simulink model "robocup_simu"  (R2022b)
settings: Solver=VariableStepAuto  StartTime=0.0  StopTime=10.0  RelTol=1e-3
values from neighbouring files (symbols this model uses):
  alpha_cap = 30    [Robotcup_V0.m]
  reduction_roues = 2.75    [Robotcup_V0.m]
  roues = 0.05    [Robotcup_V0.m]
  scaling = 31.42    [Robotcup_V0.m]
  Te = 0.100    (= 0.1)    [Robotcup_V0.m]
  u_max = 10    [Robotcup_V0.m]
  vcap = 3.2    [Robotcup_V0.m]
libraries: simulink x4
settings Model: Creator=arman  LastModifiedBy=arman

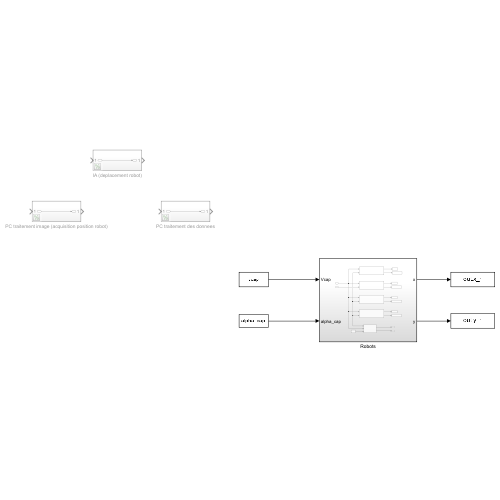
[thumbnail: Simulink's stored preview of the top-level diagram]
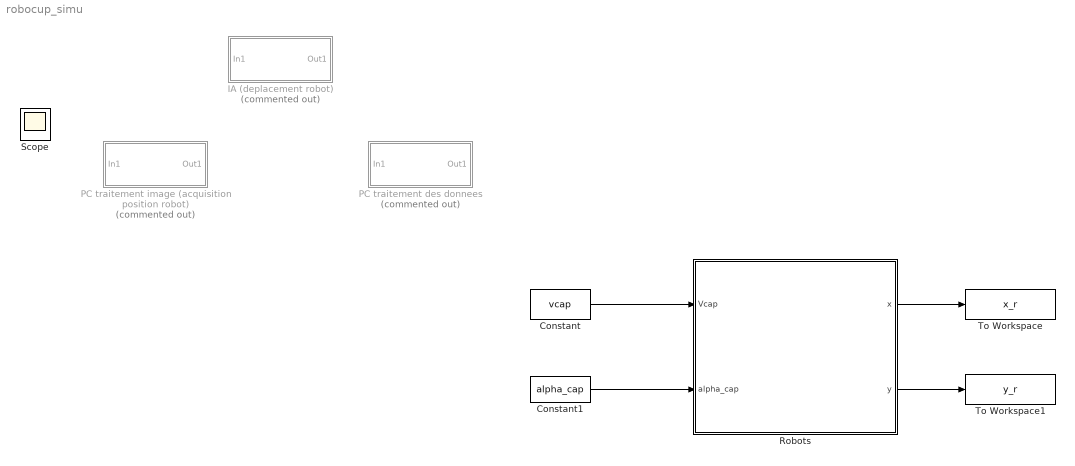
== system robocup_simu ==
  Constant : Constant  Value=vcap
  Constant1 : Constant  Value=alpha_cap
  IA (deplacement robot) : Subsystem  Commented=on
  PC traitement des donnees : Subsystem  Commented=on
  PC traitement image (acquisition position robot) : Subsystem  Commented=on
  Robots : Subsystem
  To Workspace : ToWorkspace  VariableName=x_r  SampleTime=-1
  To Workspace1 : ToWorkspace  VariableName=y_r  SaveFormat=Timeseries  SampleTime=-1
  Scope : Scope
  wires:
  Robots/1(x) -> To Workspace/1
  Robots/2(y) -> To Workspace1/1
  Constant/1 -> Robots/1(Vcap)
  Constant1/1 -> Robots/2(alpha_cap)

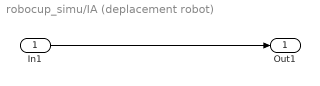
== system robocup_simu/IA (deplacement robot) ==
  In1 : Inport
  Out1 : Outport
  wires:
  In1/1 -> Out1/1

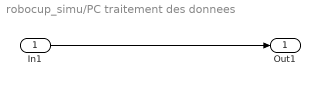
== system robocup_simu/PC traitement des donnees ==
  In1 : Inport
  Out1 : Outport
  wires:
  In1/1 -> Out1/1

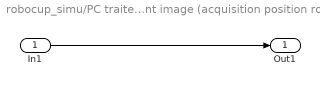
== system robocup_simu/PC traitement image (acquisition position robot) ==
  In1 : Inport
  Out1 : Outport
  wires:
  In1/1 -> Out1/1

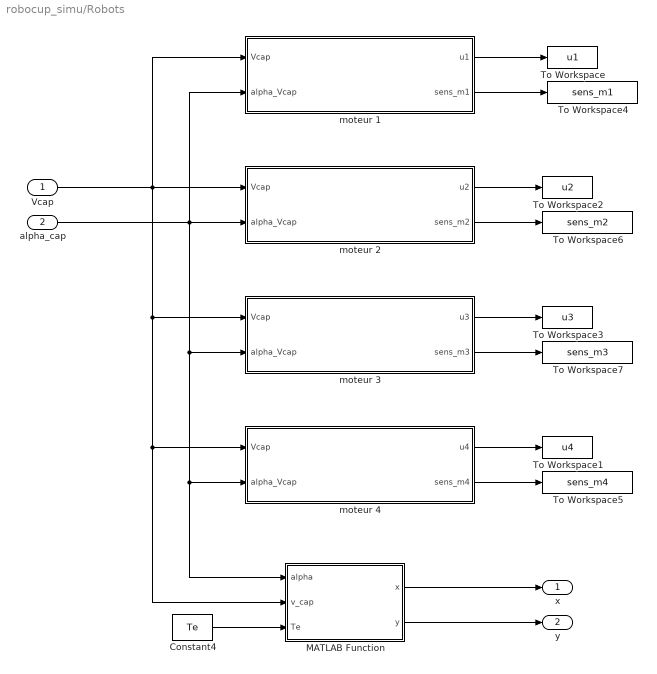
== system robocup_simu/Robots ==
  Vcap : Inport
  alpha_cap : Inport  Port=2
  Constant4 : Constant  Value=Te
  MATLAB Function : MATLAB Function  TreatAsAtomicUnit=on
  To Workspace : ToWorkspace  VariableName=u1  SaveFormat=Timeseries  SampleTime=-1
  To Workspace1 : ToWorkspace  VariableName=u4  SaveFormat=Timeseries  SampleTime=-1
  To Workspace2 : ToWorkspace  VariableName=u2  SaveFormat=Timeseries  SampleTime=-1
  To Workspace3 : ToWorkspace  VariableName=u3  SaveFormat=Timeseries  SampleTime=-1
  To Workspace4 : ToWorkspace  VariableName=sens_m1  SaveFormat=Timeseries  SampleTime=-1
  To Workspace5 : ToWorkspace  VariableName=sens_m4  SaveFormat=Timeseries  SampleTime=-1
  To Workspace6 : ToWorkspace  VariableName=sens_m2  SaveFormat=Timeseries  SampleTime=-1
  To Workspace7 : ToWorkspace  VariableName=sens_m3  SaveFormat=Timeseries  SampleTime=-1
  moteur 1 : Subsystem
  moteur 2 : Subsystem
  moteur 3 : Subsystem
  moteur 4 : Subsystem
  x : Outport
  y : Outport  Port=2
  wires:
  moteur 3/1(u3) -> To Workspace3/1
  moteur 2/1(u2) -> To Workspace2/1
  moteur 1/1(u1) -> To Workspace/1
  moteur 4/1(u4) -> To Workspace1/1
  moteur 1/2(sens_m1) -> To Workspace4/1
  moteur 3/2(sens_m3) -> To Workspace7/1
  moteur 2/2(sens_m2) -> To Workspace6/1
  moteur 4/2(sens_m4) -> To Workspace5/1
  MATLAB Function/2(y) -> y/1
  MATLAB Function/1(x) -> x/1
  Vcap/1 -> MATLAB Function/2(v_cap), moteur 4/1(Vcap), moteur 3/1(Vcap), moteur 2/1(Vcap), moteur 1/1(Vcap)
  alpha_cap/1 -> MATLAB Function/1(alpha), moteur 4/2(alpha_Vcap), moteur 3/2(alpha_Vcap), moteur 1/2(alpha_Vcap), moteur 2/2(alpha_Vcap)
  Constant4/1 -> MATLAB Function/3(Te)

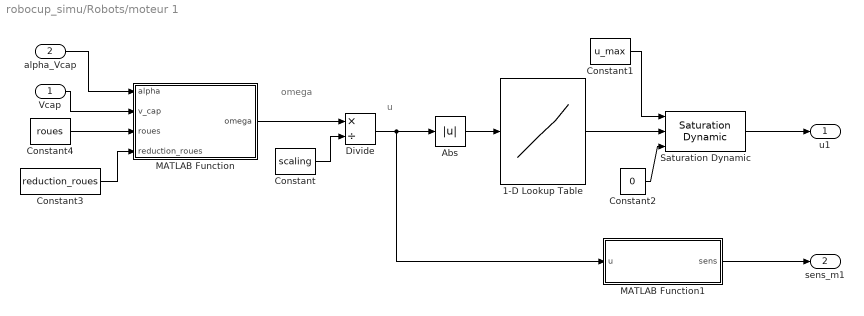
== system robocup_simu/Robots/moteur 1 ==
  note: omega
  note: u
  Vcap : Inport
  alpha_Vcap : Inport  Port=2
  1-D Lookup Table : Lookup_n-D  NumberOfTableDimensions=1  BreakpointsForDimension1=[0 0.16 0.17 0.32 0.33 1 1.5 2 3 4 10]  Table=[0 0 0.25 0.25 0.33 1 1.5 2 3 4 10]  InternalRulePriority=Speed  RndMeth=Simplest
  Abs : Abs  SaturateOnIntegerOverflow=off
  Constant : Constant  Value=scaling
  Constant1 : Constant  Value=u_max
  Constant2 : Constant  Value=0
  Constant3 : Constant  Value=reduction_roues
  Constant4 : Constant  Value=roues
  Divide : Product  Inputs=*/
  MATLAB Function : MATLAB Function  TreatAsAtomicUnit=on
  MATLAB Function1 : MATLAB Function  TreatAsAtomicUnit=on
  Saturation Dynamic : simulink/Discontinuities/Saturation Dynamic  OutMin=[]  OutMax=[]  OutDataTypeStr=Inherit: Same as second input  OutDataType=fixdt(1, 16)  OutScaling=2^-10  DoSatur=off
  u1 : Outport
  sens_m1 : Outport  Port=2
  wires:
  MATLAB Function/1(omega) -> Divide/1
  Constant/1 -> Divide/2
  Constant1/1 -> Saturation Dynamic/1
  Constant2/1 -> Saturation Dynamic/3
  Divide/1 -> MATLAB Function1/1(u), Abs/1
  Abs/1 -> 1-D Lookup Table/1
  1-D Lookup Table/1 -> Saturation Dynamic/2
  Saturation Dynamic/1 -> u1/1
  MATLAB Function1/1(sens) -> sens_m1/1
  Constant4/1 -> MATLAB Function/3(roues)
  Vcap/1 -> MATLAB Function/2(v_cap)
  Constant3/1 -> MATLAB Function/4(reduction_roues)
  alpha_Vcap/1 -> MATLAB Function/1(alpha)

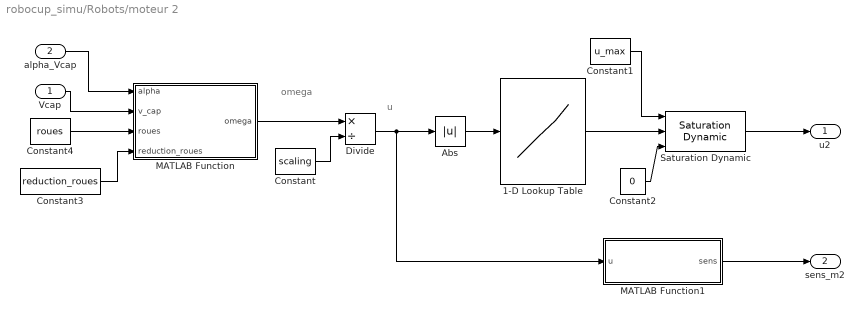
== system robocup_simu/Robots/moteur 2 ==
  note: omega
  note: u
  Vcap : Inport
  alpha_Vcap : Inport  Port=2
  1-D Lookup Table : Lookup_n-D  NumberOfTableDimensions=1  BreakpointsForDimension1=[0 0.16 0.17 0.32 0.33 1 1.5 2 3 4 10]  Table=[0 0 0.25 0.25 0.33 1 1.5 2 3 4 10]  InternalRulePriority=Speed  RndMeth=Simplest
  Abs : Abs  SaturateOnIntegerOverflow=off
  Constant : Constant  Value=scaling
  Constant1 : Constant  Value=u_max
  Constant2 : Constant  Value=0
  Constant3 : Constant  Value=reduction_roues
  Constant4 : Constant  Value=roues
  Divide : Product  Inputs=*/
  MATLAB Function : MATLAB Function  TreatAsAtomicUnit=on
  MATLAB Function1 : MATLAB Function  TreatAsAtomicUnit=on
  Saturation Dynamic : simulink/Discontinuities/Saturation Dynamic  OutMin=[]  OutMax=[]  OutDataTypeStr=Inherit: Same as second input  OutDataType=fixdt(1, 16)  OutScaling=2^-10  DoSatur=off
  u2 : Outport
  sens_m2 : Outport  Port=2
  wires:
  MATLAB Function/1(omega) -> Divide/1
  Constant/1 -> Divide/2
  Constant1/1 -> Saturation Dynamic/1
  Constant2/1 -> Saturation Dynamic/3
  Divide/1 -> MATLAB Function1/1(u), Abs/1
  Abs/1 -> 1-D Lookup Table/1
  1-D Lookup Table/1 -> Saturation Dynamic/2
  Saturation Dynamic/1 -> u2/1
  MATLAB Function1/1(sens) -> sens_m2/1
  Constant4/1 -> MATLAB Function/3(roues)
  Vcap/1 -> MATLAB Function/2(v_cap)
  Constant3/1 -> MATLAB Function/4(reduction_roues)
  alpha_Vcap/1 -> MATLAB Function/1(alpha)

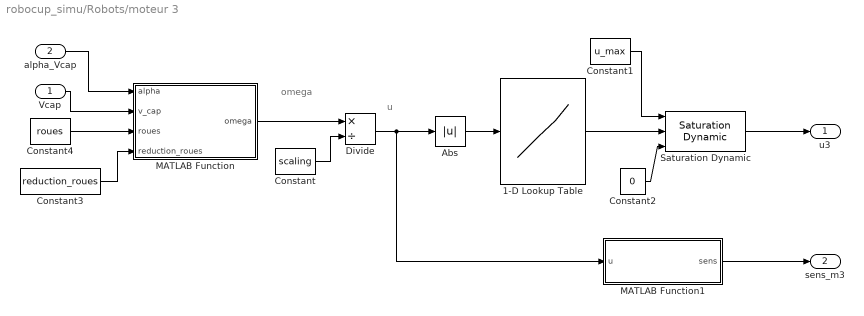
== system robocup_simu/Robots/moteur 3 ==
  note: omega
  note: u
  Vcap : Inport
  alpha_Vcap : Inport  Port=2
  1-D Lookup Table : Lookup_n-D  NumberOfTableDimensions=1  BreakpointsForDimension1=[0 0.16 0.17 0.32 0.33 1 1.5 2 3 4 10]  Table=[0 0 0.25 0.25 0.33 1 1.5 2 3 4 10]  InternalRulePriority=Speed  RndMeth=Simplest
  Abs : Abs  SaturateOnIntegerOverflow=off
  Constant : Constant  Value=scaling
  Constant1 : Constant  Value=u_max
  Constant2 : Constant  Value=0
  Constant3 : Constant  Value=reduction_roues
  Constant4 : Constant  Value=roues
  Divide : Product  Inputs=*/
  MATLAB Function : MATLAB Function  TreatAsAtomicUnit=on
  MATLAB Function1 : MATLAB Function  TreatAsAtomicUnit=on
  Saturation Dynamic : simulink/Discontinuities/Saturation Dynamic  OutMin=[]  OutMax=[]  OutDataTypeStr=Inherit: Same as second input  OutDataType=fixdt(1, 16)  OutScaling=2^-10  DoSatur=off
  u3 : Outport
  sens_m3 : Outport  Port=2
  wires:
  MATLAB Function/1(omega) -> Divide/1
  Constant/1 -> Divide/2
  Constant1/1 -> Saturation Dynamic/1
  Constant2/1 -> Saturation Dynamic/3
  Divide/1 -> MATLAB Function1/1(u), Abs/1
  Abs/1 -> 1-D Lookup Table/1
  1-D Lookup Table/1 -> Saturation Dynamic/2
  Saturation Dynamic/1 -> u3/1
  MATLAB Function1/1(sens) -> sens_m3/1
  Constant4/1 -> MATLAB Function/3(roues)
  Vcap/1 -> MATLAB Function/2(v_cap)
  Constant3/1 -> MATLAB Function/4(reduction_roues)
  alpha_Vcap/1 -> MATLAB Function/1(alpha)

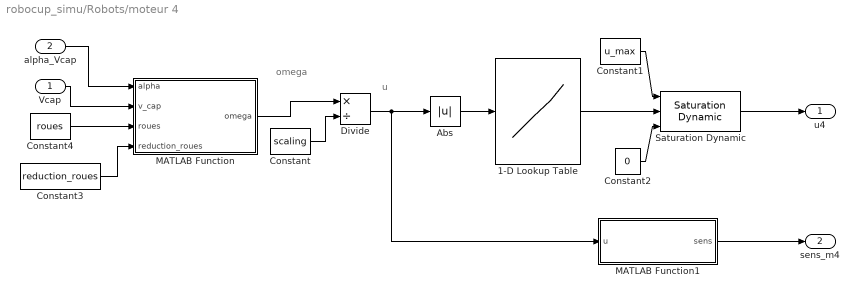
== system robocup_simu/Robots/moteur 4 ==
  note: omega
  note: u
  Vcap : Inport
  alpha_Vcap : Inport  Port=2
  1-D Lookup Table : Lookup_n-D  NumberOfTableDimensions=1  BreakpointsForDimension1=[0 0.16 0.17 0.32 0.33 1 1.5 2 3 4 10]  Table=[0 0 0.25 0.25 0.33 1 1.5 2 3 4 10]  InternalRulePriority=Speed  RndMeth=Simplest
  Abs : Abs  SaturateOnIntegerOverflow=off
  Constant : Constant  Value=scaling
  Constant1 : Constant  Value=u_max
  Constant2 : Constant  Value=0
  Constant3 : Constant  Value=reduction_roues
  Constant4 : Constant  Value=roues
  Divide : Product  Inputs=*/
  MATLAB Function : MATLAB Function  TreatAsAtomicUnit=on
  MATLAB Function1 : MATLAB Function  TreatAsAtomicUnit=on
  Saturation Dynamic : simulink/Discontinuities/Saturation Dynamic  OutMin=[]  OutMax=[]  OutDataTypeStr=Inherit: Same as second input  OutDataType=fixdt(1, 16)  OutScaling=2^-10  DoSatur=off
  u4 : Outport
  sens_m4 : Outport  Port=2
  wires:
  alpha_Vcap/1 -> MATLAB Function/1(alpha)
  Vcap/1 -> MATLAB Function/2(v_cap)
  MATLAB Function/1(omega) -> Divide/1
  Constant/1 -> Divide/2
  Constant1/1 -> Saturation Dynamic/1
  Constant2/1 -> Saturation Dynamic/3
  Divide/1 -> MATLAB Function1/1(u), Abs/1
  Abs/1 -> 1-D Lookup Table/1
  1-D Lookup Table/1 -> Saturation Dynamic/2
  Saturation Dynamic/1 -> u4/1
  MATLAB Function1/1(sens) -> sens_m4/1
  Constant3/1 -> MATLAB Function/4(reduction_roues)
  Constant4/1 -> MATLAB Function/3(roues)

== matlab function robocup_simu/Robots/moteur 1/MATLAB Function1 ==
  data: u input; sens output
function sens = fcn(u)

if (u < 0)
    sens = 0;  %CW
else
    sens = 1;  %CCW
end

== matlab function robocup_simu/Robots/moteur 1/MATLAB Function ==
  data: alpha input; omega output; v_cap input; roues input; reduction_roues input
function omega = fcn(alpha,v_cap,roues,reduction_roues)

omega = (1/roues) * v_cap * cos((45-alpha)*pi/180)* reduction_roues;

== matlab function robocup_simu/Robots/moteur 2/MATLAB Function ==
  data: alpha input; omega output; v_cap input; roues input; reduction_roues input
function omega = fcn(alpha,v_cap,roues,reduction_roues)

omega = (1/roues) * v_cap * cos((45+alpha)*pi/180)* reduction_roues;

== matlab function robocup_simu/Robots/moteur 2/MATLAB Function1 ==
  data: u input; sens output
function sens = fcn(u)

if (u < 0)
    sens = 1;  %CCW
else
    sens = 0;  %CW
end

== matlab function robocup_simu/Robots/moteur 3/MATLAB Function ==
  data: alpha input; omega output; v_cap input; roues input; reduction_roues input
function omega = fcn(alpha,v_cap,roues,reduction_roues)

omega = (1/roues) * v_cap * cos((45-alpha)*pi/180)* reduction_roues;

== matlab function robocup_simu/Robots/moteur 3/MATLAB Function1 ==
  data: u input; sens output
function sens = fcn(u)

if (u < 0)
    sens = 1;  %CCW
else
    sens = 0;  %CW
end

== matlab function robocup_simu/Robots/moteur 4/MATLAB Function ==
  data: alpha input; omega output; v_cap input; roues input; reduction_roues input
function omega = fcn(alpha,v_cap,roues,reduction_roues)

omega = (1/roues) * v_cap * cos((45+alpha)*pi/180)* reduction_roues;

== matlab function robocup_simu/Robots/moteur 4/MATLAB Function1 ==
  data: u input; sens output
function sens = fcn(u)

if (u < 0)
    sens = 0;  %CW
else
    sens = 1;  %CCW
end

== matlab function robocup_simu/Robots/MATLAB Function ==
  data: alpha input; x output; v_cap input; y output; Te input
function [x,y] = fcn(alpha,v_cap,Te)

x = Te * cos(alpha) * v_cap;
y = Te * sin(alpha) * v_cap;
